simulink model "LinearizedPlant"  (R2024b)
settings: Solver=ode8  StartTime=0.0  StopTime=60  FixedStep=0.0001  RelTol=1e-3
libraries: simulink_extras x2, aerolibactuator x1
settings Model: Creator=jonno  LastModifiedBy=jonno

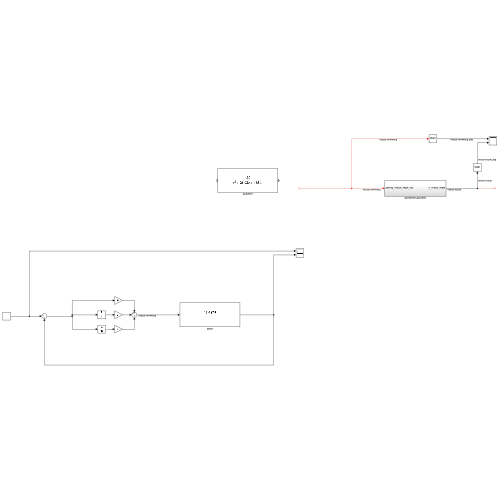
[thumbnail: Simulink's stored preview of the top-level diagram]
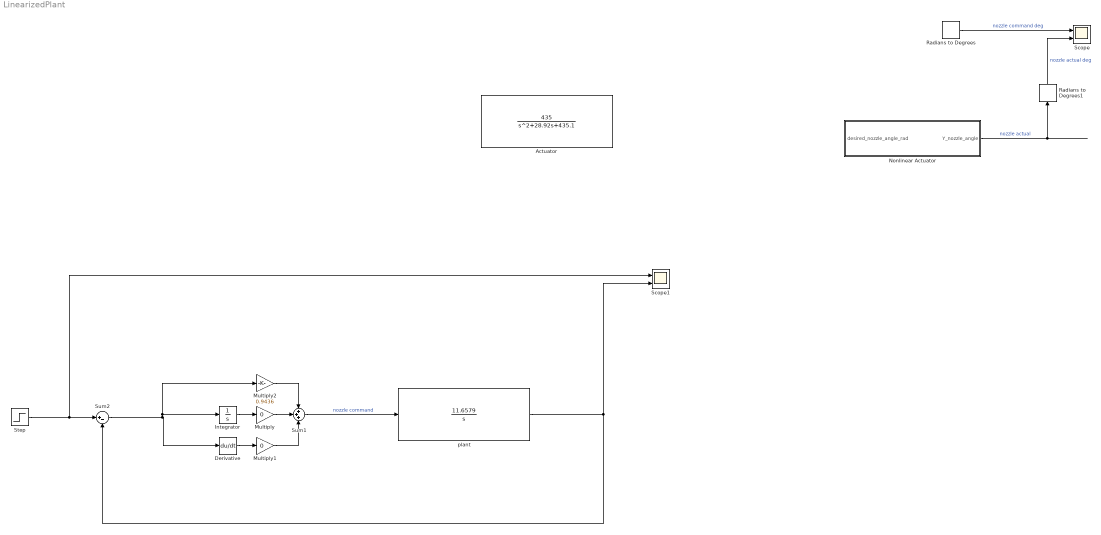
== system LinearizedPlant ==
  Actuator : TransferFcn  Numerator=[435]  Denominator="[1  28.92 435.1]"
  Derivative : Derivative
  Integrator : Integrator
  Multiply : Gain  Gain=0
  Multiply1 : Gain  Gain=0
  Multiply2 : Gain  Gain=0.9436
  Nonlinear Actuator : Subsystem
  Radians to Degrees : simulink_extras/Transformations/Radians to Degrees
  Radians to Degrees1 : simulink_extras/Transformations/Radians to Degrees
  Scope : Scope  NumInputPorts=2
  Scope1 : Scope  NumInputPorts=2
  Step : Step  After=30*pi/180  SampleTime=0
  Sum1 : Sum  Inputs=+++
  Sum2 : Sum  Inputs=|+-
  plant : TransferFcn  Numerator=[11.6579]  Denominator=[1 0]
  wires:
  Sum2/1 -> Integrator/1, Multiply2/1, Derivative/1
  Integrator/1 -> Multiply/1
  Derivative/1 -> Multiply1/1
  Multiply/1 -> Sum1/2
  Multiply1/1 -> Sum1/3
  Multiply2/1 -> Sum1/1
  plant/1 -> Sum2/2, Scope1/2
  Step/1 -> Scope1/1, Sum2/1
  Radians to Degrees1/1 -> Scope/2  "nozzle actual deg"
  Nonlinear Actuator/1(Y_nozzle_angle) -> Radians to Degrees1/1  "nozzle actual"
  Radians to Degrees/1 -> Scope/1  "nozzle command deg"
  ? -> Nonlinear Actuator/1(desired_nozzle_angle_rad), Radians to Degrees/1  "nozzle command"
  Sum1/1 -> plant/1  "nozzle command"

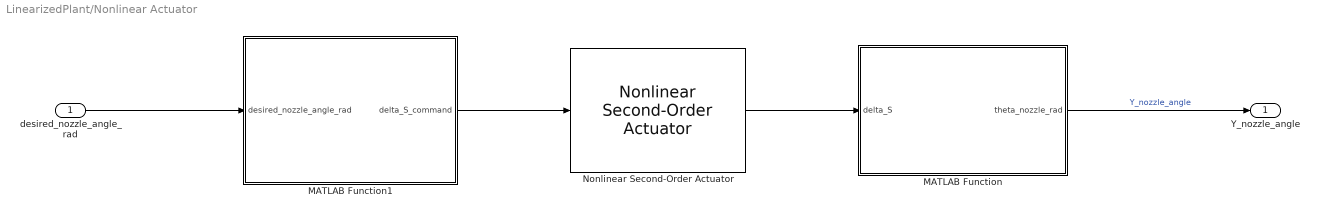
== system LinearizedPlant/Nonlinear Actuator ==
  desired_nozzle_angle_rad : Inport
  MATLAB Function : MATLAB Function  TreatAsAtomicUnit=on
  MATLAB Function1 : MATLAB Function  TreatAsAtomicUnit=on
  Nonlinear Second-Order Actuator : aerolibactuator/Nonlinear Second-Order Actuator  wn_fin=27  z_fin=0.7  fin_max=0.035  fin_min=-0.035  fin_maxrate=0.133  fin_act_0=0  fin_act_vel=0
  Y_nozzle_angle : Outport
  wires:
  MATLAB Function/1(theta_nozzle_rad) -> Y_nozzle_angle/1  "Y_nozzle_angle"
  MATLAB Function1/1(delta_S_command) -> Nonlinear Second-Order Actuator/1
  desired_nozzle_angle_rad/1 -> MATLAB Function1/1(desired_nozzle_angle_rad)
  Nonlinear Second-Order Actuator/1 -> MATLAB Function/1(delta_S)

== matlab function LinearizedPlant/Nonlinear Actuator/MATLAB Function ==
  data: delta_S input; theta_nozzle_rad output
function theta_nozzle_rad = linkage_to_nozzle_angle(delta_S)
% Calculates nozzle angle deflection based on linear actuator displacement (delta_S).
% Assumes delta_S is the change in length from the initial actuator length S0.
% theta_nozzle_rad is the CHANGE in the angle between linkage arms from their initial configuration.
% Input delta_S is expected in meters.
% Output theta_nozzle_rad is in radians.

%#codegen % Required for Simulink code generation

% Linkage parameters (constants)
l = 0.173086;   % m (First arm length)
r = 0.187926;   % m (Second arm length)
S0 = 0.221779;  % m (Initial actuator length when theta_nozzle_rad is defined as 0)

% --- Calculate the initial internal angle based on S0, l, and r ---
% This is the angle between arms l and r when delta_S = 0.
% cos(initial_internal_angle) = (l^2 + r^2 - S0^2) / (2 * l * r)
cos_arg_initial = (l^2 + r^2 - S0^2) / (2 * l * r);

% Clamp for safety, though with consistent S0, l, r, it should be valid
if cos_arg_initial > 1.0
    cos_arg_initial = 1.0;
elseif cos_arg_initial < -1.0
    cos_arg_initial = -1.0;
end
initial_internal_angle_rad = acos(cos_arg_initial);
% --------------------------------------------------------------------

% Calculate current total actuator length
S_current = S0 + delta_S;

% Calculate the argument for acos for the CURRENT internal angle
% cos(current_internal_angle) = (l^2 + r^2 - S_current^2) / (2 * l * r)
cos_arg_current = (l^2 + r^2 - S_current^2) / (2 * l * r);

% Clamp cos_arg_current to the valid range [-1, 1]
if cos_arg_current > 1.0
    cos_arg_current = 1.0;
elseif cos_arg_current < -1.0
    cos_arg_current = -1.0;
end

% Calculate current internal angle between arms l and r
current_internal_angle_rad = acos(cos_arg_current); % Result is in radians

% Calculate theta_nozzle_rad as the CHANGE from the initial internal angle
theta_nozzle_rad = current_internal_angle_rad - initial_internal_angle_rad;

% --- Optional: Map this change in internal angle to actual nozzle orientation ---
% If the nozzle's zero position (theta_nozzle_rad = 0) corresponds to a specific
% absolute orientation (e.g., aligned with rocket body), and 'alpha_deg' from your
% original code represented some offset or component of the initial nozzle orientation,
% you might need an additional step.
% For example, if alpha_deg was an offset:
% nozzle_absolute_angle_rad = theta_nozzle_rad + (alpha_deg_from_original_code * pi/180);
% But based on your problem description, the current theta_nozzle_rad (as a change)
% is likely what's needed if delta_S=0 should give theta_nozzle_rad=0.
end

== matlab function LinearizedPlant/Nonlinear Actuator/MATLAB Function1 ==
  data: desired_nozzle_angle_rad input; delta_S_command output
function delta_S_command = inverse_kinematics_nozzle(desired_nozzle_angle_rad)
% Calculates the required linear actuator stroke (delta_S) for a desired
% nozzle deflection angle (desired_nozzle_angle_rad).
% desired_nozzle_angle_rad is the CHANGE in the angle between linkage arms
% from their initial configuration (when delta_S = 0).
%
% Input:
%   desired_nozzle_angle_rad: The desired change in nozzle angle, in RADIANS.
%
% Output:
%   delta_S_command: The required change in actuator length (stroke), in meters.

%#codegen % Required for Simulink code generation

% Linkage parameters (constants)
l = 0.173086;   % m (First arm length)
r = 0.187926;   % m (Second arm length)
S0 = 0.221779;  % m (Initial actuator length when desired_nozzle_angle_rad is 0)

% --- Calculate the initial internal angle based on S0, l, and r ---
% This is the angle between arms l and r when desired_nozzle_angle_rad is 0 (and delta_S is 0).
% cos(initial_internal_angle) = (l^2 + r^2 - S0^2) / (2 * l * r)
cos_arg_initial = (l^2 + r^2 - S0^2) / (2 * l * r);

% Clamp for safety, though with consistent S0, l, r, it should be valid
if cos_arg_initial > 1.0
    cos_arg_initial = 1.0;
elseif cos_arg_initial < -1.0
    cos_arg_initial = -1.0;
end
initial_internal_angle_rad = acos(cos_arg_initial);
% --------------------------------------------------------------------

% Calculate the target total internal angle for the linkage
% This is the initial angle PLUS the desired change.
target_total_internal_angle_rad = initial_internal_angle_rad + desired_nozzle_angle_rad;

% Calculate S_total_squared = (S0 + delta_S)^2 using the law of cosines
% for the target_total_internal_angle_rad
S_total_squared = l^2 + r^2 - 2*l*r*cos(target_total_internal_angle_rad);

% --- Handle Physical Impossibility (Saturation) ---
% S_total_squared should theoretically be between (l-r)^2 and (l+r)^2.
% (l-r)^2 corresponds to the arms being collinear and extended in opposite directions (shortest S).
% (l+r)^2 corresponds to the arms being collinear and extended in the same direction (longest S).
S_min_possible_squared = (l-r)^2;
S_max_possible_squared = (l+r)^2;

if S_total_squared < S_min_possible_squared
    % This can happen if target_total_internal_angle_rad is too close to 0 or pi (collinear)
    % and the desired S is shorter than physically possible.
    % Or due to floating point errors if very close to the limit.
    coder.varsize('warning_text_min', [1, 200]);
    warning_text_min = sprintf('Warning: Desired angle (%.2f rad from initial) leads to S_total_squared (%.4e) < S_min_possible_squared (%.4e). Clamping.', desired_nozzle_angle_rad, S_total_squared, S_min_possible_squared);
    warning(warning_text_min);
    S_total_squared = S_min_possible_squared;
elseif S_total_squared > S_max_possible_squared
    % This implies the angle is such that it requires S > l+r, which is impossible.
    coder.varsize('warning_text_max', [1, 200]);
    warning_text_max = sprintf('Warning: Desired angle (%.2f rad from initial) leads to S_total_squared (%.4e) > S_max_possible_squared (%.4e). Clamping.', desired_nozzle_angle_rad, S_total_squared, S_max_possible_squared);
    warning(warning_text_max);
    S_total_squared = S_max_possible_squared;
end
% An additional check if S_total_squared somehow still ended up negative, though the above should prevent it.
if S_total_squared < 0
    S_total_squared = 0; % Fallback, should ideally be S_min_possible_squared
end
% --- End Handle Physical Impossibility ---

% Calculate the total desired actuator length S_total = S0 + delta_S
S_total_desired = sqrt(S_total_squared);

% Calculate the required actuator stroke delta_S
delta_S_command = S_total_desired - S0;

end
